simulink model "closedloop"  (Simulink 10.0)
settings: Solver=ode45  StartTime=0.0  StopTime=1000  RelTol=1e-10  AbsTol=1e-10
libraries: cstblocks x2
settings Model: Creator=horch  LastModifiedBy=bianc  ExtModeTrigMode=oneshot  ExtModeArmWhenConnect=off
settings SolverCC: AutoScaleAbsTol=off
settings DataIOCC: SignalLoggingSaveFormat=ModelDataLogs
settings OptimizationCC: BooleanDataType=off
settings DebuggingCC: SaveWithParameterizedLinksMsg=none  SignalResolutionControl=TryResolveAllWithWarning  MultiTaskDSMMsg=warning  MultiTaskCondExecSysMsg=none
settings HardwareCC: TargetUnknown=on
settings GRTTargetCC: GeneratePreprocessorConditionals=Disable all
settings ConfigComp: CovExternalEMLEnable=off

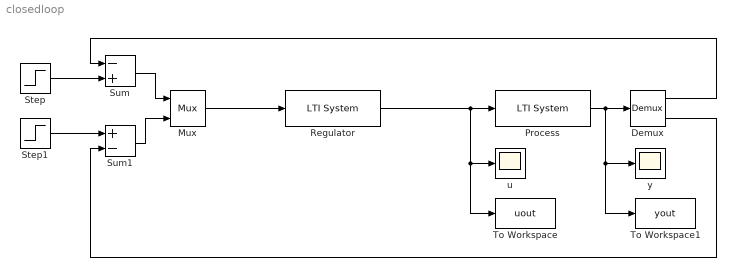
== system closedloop ==
  Demux : Demux  Outputs=2
  Mux : Mux  Inputs=2
  Process : cstblocks/LTI System  sys=G_nonmp  IC=0
  Regulator : cstblocks/LTI System  sys=F  IC=0
  Step : Step  Time=100  SampleTime=0
  Step1 : Step  Time=500  SampleTime=0
  Sum : Sum  Inputs=-+  SaturateOnIntegerOverflow=on  InputSameDT=on  OutDataTypeStr=Inherit: Same as first input
  Sum1 : Sum  Inputs=+-  SaturateOnIntegerOverflow=on  InputSameDT=on  OutDataTypeStr=Inherit: Same as first input
  To Workspace : ToWorkspace  VariableName=uout  SaveFormat=Timeseries  SampleTime=-1
  To Workspace1 : ToWorkspace  VariableName=yout  SaveFormat=Timeseries  SampleTime=-1
  u : Scope
  y : Scope
  wires:
  Mux/1 -> Regulator/1
  Step/1 -> Sum/2
  Demux/1 -> Sum/1
  Demux/2 -> Sum1/2
  Process/1 -> Demux/1, y/1, To Workspace1/1
  Step1/1 -> Sum1/1
  Sum/1 -> Mux/1
  Sum1/1 -> Mux/2
  Regulator/1 -> Process/1, To Workspace/1, u/1
